simulink model "manifold_blocks"  (R2022b)
settings: Solver=ode45  StartTime=0.0  StopTime=10.0  MaxStep=0.2  RelTol=1e-3  EnableMultiTasking=on
InitFcn:
  | % Input data
  | load manifold_press_start.mat
settings Model: Creator=dlange  LastModifiedBy=bensweet
settings SolverCC: AlgebraicLoopSolver=TrustRegion
settings DataIOCC: ExternalInput=[t, mdot_in, w]  LimitDataPoints=on  LoadExternalInput=on  SaveFormat=Array  ReturnWorkspaceOutputs=off
settings OptimizationCC: ExpressionDepthLimit=2147483647  InitFltsAndDblsToZero=on  LifeSpan=inf
settings DebuggingCC: UnconnectedInputMsg=warning  UnconnectedOutputMsg=warning  UnconnectedLineMsg=warning  PregeneratedLibrarySubsystemCodeDiagnostic=none  SFMachineParentedDataDiag=warning
settings HardwareCC: ProdBitPerPointer=32  ProdBitPerSizeT=32  ProdBitPerPtrDiffT=32  ProdLargestAtomicFloat=None  ProdIntDivRoundTo=Undefined  ProdEndianess=Unspecified  ProdWordSize=32  ProdHWDeviceType=32-bit Generic
settings ModelReferenceCC: EnableRefExpFcnMdlSchedulingChecks=on  PropagateSignalLabelsOutOfModel=off
settings SFSimCC: SimUseLocalCustomCode=off
settings RTWCC: RTWUseLocalCustomCode=off  DLArmComputeVersion=19.05
settings CodeAppCC: StateflowObjectComments=on
settings GRTTargetCC: TargetFcnLib=ansi_tfl_tmw.mat  TargetLangStandard=C89/C90 (ANSI)  CombineOutputUpdateFcns=off  GRTInterface=on
settings ConfigComp: CovMetricSettings=dw  CovSaveCumulativeToWorkspaceVar=on  CovSaveSingleToWorkspaceVar=on  CovExternalEMLEnable=off  CovSFcnEnable=off

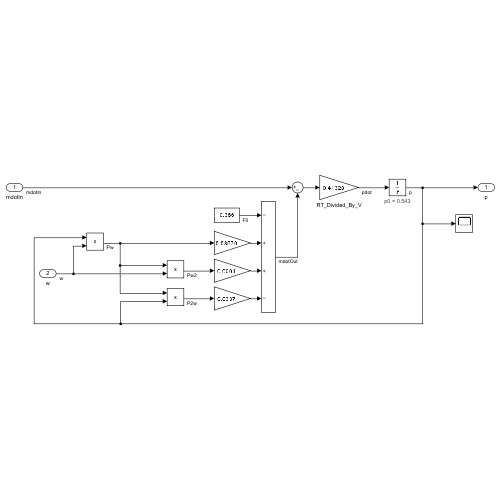
[thumbnail: Simulink's stored preview of the top-level diagram]
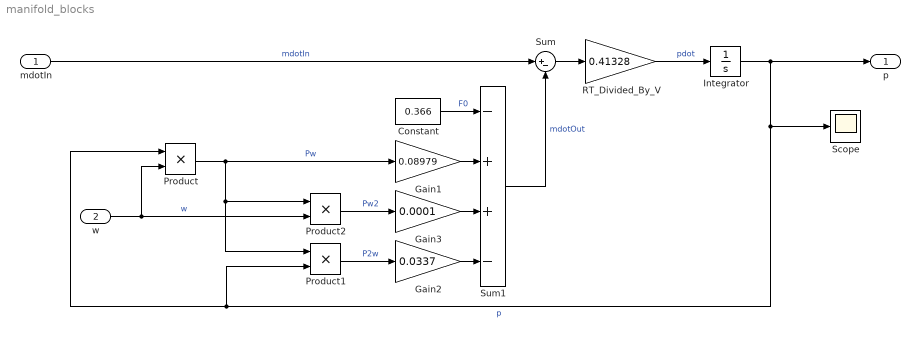
== system manifold_blocks ==
  mdotIn : Inport
  w : Inport  Port=2
  Constant : Constant  Value=0.366
  Gain1 : Gain  Gain=0.08979
  Gain2 : Gain  Gain=0.0337
  Gain3 : Gain  Gain=0.0001
  Integrator : Integrator  InitialCondition=0.543
      settings: AttributesFormatString=p0 = %<InitialCondition>
  Product : Product  RndMeth=Zero
  Product1 : Product  RndMeth=Zero
  Product2 : Product  RndMeth=Zero
  RT_Divided_By_V : Gain  Gain=0.41328
  Scope : Scope
  Sum : Sum  Inputs=|+-
  Sum1 : Sum  Inputs=-++-
  p : Outport  VectorParamsAs1DForOutWhenUnconnected=off
  wires:
  Integrator/1 -> p/1, Scope/1, Product/1, Product1/2  "p"
  RT_Divided_By_V/1 -> Integrator/1  "pdot"
  mdotIn/1 -> Sum/1  "mdotIn"
  Sum/1 -> RT_Divided_By_V/1
  Constant/1 -> Sum1/1  "F0"
  Gain1/1 -> Sum1/2
  Product/1 -> Gain1/1, Product1/1, Product2/1  "Pw"
  Product1/1 -> Gain2/1  "P2w"
  Product2/1 -> Gain3/1  "Pw2"
  Sum1/1 -> Sum/2  "mdotOut"
  Gain3/1 -> Sum1/3
  Gain2/1 -> Sum1/4
  w/1 -> Product/2, Product2/2  "w"
